simulink model "inverted_pendulum_kalman"  (R2016b)
settings: Solver=VariableStepAuto  StartTime=0.0  StopTime=10  RelTol=1e-3
settings Model: Creator=Quy  LastModifiedBy=Anass

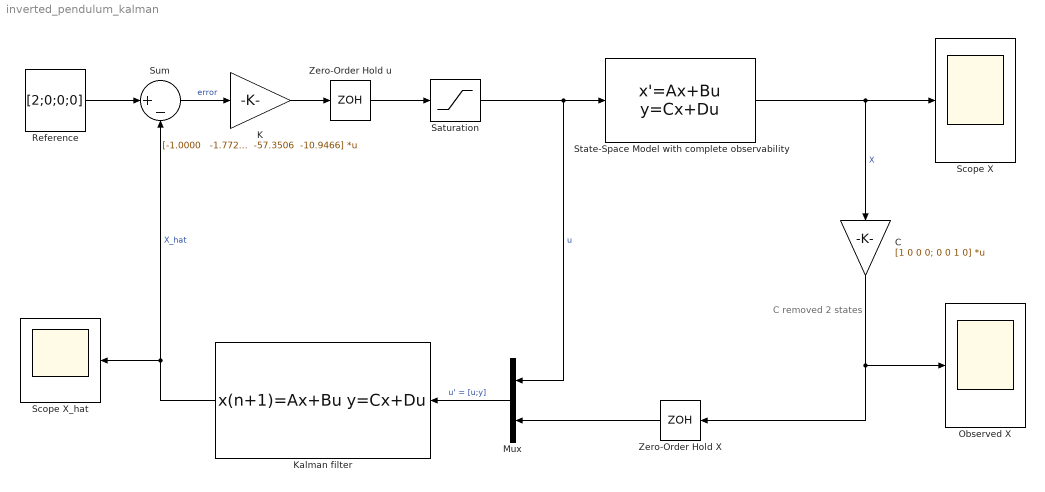
== system inverted_pendulum_kalman ==
  note: C removed 2 states
  C : Gain  Gain=[1 0 0 0; 0 0 1 0]  Multiplication=Matrix(K*u) (u vector)
  K : Gain  Gain="[-1.0000   -1.7726  -57.3506  -10.9466]"  Multiplication=Matrix(K*u) (u vector)
  Kalman filter : DiscreteStateSpace  A=|  B=|  C=eye(4)  D=zeros(4,3)  X0=[1;0;0;0]  SampleTime=0.01  StateIdentifier=X_hat
      A=|
      | [    0.9696    0.0100    0.0007         0;
      |    -0.0461    0.8959    0.0098         0;
      |     0.0007         0    0.8846    0.0100;
      |     0.0000    0.0431   -0.2989    0.9938]
      B=|
      | [         0    0.0304   -0.0007;
      |     0.5129    0.0461   -0.0098;
      |          0   -0.0007    0.1154;
      |    -0.2102   -0.0000    0.6663]
  Mux : Mux  Inputs=2
  Observed X : Scope
  Reference : Constant  Value=[2;0;0;0]
  Saturation : Saturate  UpperLimit=0.9  LowerLimit=-0.8
  Scope X : Scope
  Scope X_hat : Scope
  State-Space Model with complete observability : StateSpace  A=|  B=|  C=eye(4)  D=[0;0;0;0]  X0=[1; 0; 0; 0]
      A=|
      | [0    1.0000         0         0;
      |          0  -10.4100         0         0;
      |          0         0         0    1.0000;
      |          0    4.3111   36.7400   -0.6249]
      B=|
      | [0;
      |    51.2860;
      |          0;
      |   -21.0230]
  Sum : Sum  Inputs=|+-
  Zero-Order Hold X : ZeroOrderHold  SampleTime=0.01
  Zero-Order Hold u : ZeroOrderHold  SampleTime=0.01
  wires:
  State-Space Model with complete observability/1 -> C/1, Scope X/1  "X"
  Sum/1 -> K/1  "error"
  Reference/1 -> Sum/1
  K/1 -> Zero-Order Hold u/1
  Zero-Order Hold u/1 -> Saturation/1
  Mux/1 -> Kalman filter/1  "u' = [u;y]"
  Saturation/1 -> Mux/1, State-Space Model with complete observability/1  "u"
  Kalman filter/1 -> Scope X_hat/1, Sum/2  "X_hat"
  C/1 -> Zero-Order Hold X/1, Observed X/1
  Zero-Order Hold X/1 -> Mux/2
